simulink model "w2prob4"  (R2020a)
settings: Solver=VariableStepAuto  StartTime=0.0  StopTime=10.0  RelTol=1e-3
PostLoadFcn:
  | J = 3.2284E-6;
  | b = 3.5077E-6;
  | Ke = 0.0274;
  | Kt = 0.0274;
  | R = 4;
  | L = 2.75E-6;
settings Model: DataDictionary=w2p4vars.sldd  Creator=Anjali123  LastModifiedBy=Anjali123

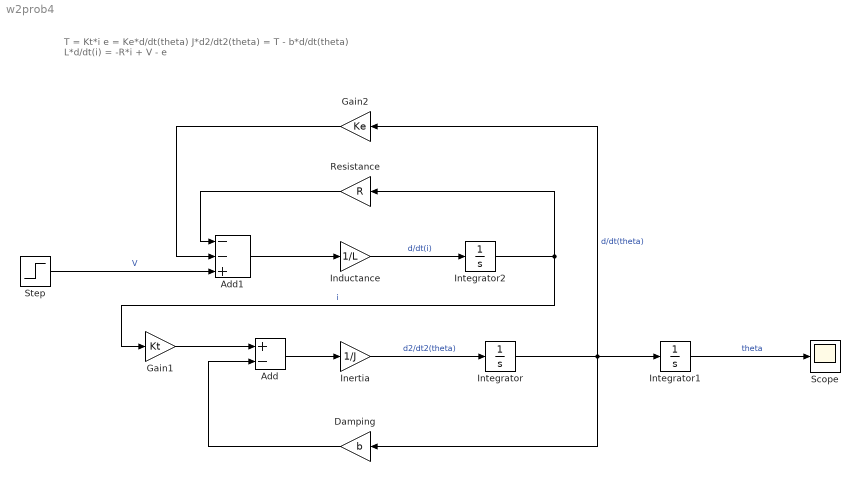
== system w2prob4 ==
  note: T = Kt*i
      | e = Ke*d/dt(theta)
      | J*d2/dt2(theta) = T - b*d/dt(theta)
      | L*d/dt(i) = -R*i + V - e
  "Add " : Sum  Inputs=+-
  "Add1 " : Sum  Inputs=--+
  Damping : Gain  Gain=b
  Gain1 : Gain  Gain=Kt
  Gain2 : Gain  Gain=Ke
  Inductance : Gain  Gain=1/L
  Inertia : Gain  Gain=1/J
  "Integrator " : Integrator
  "Integrator1 " : Integrator
  "Integrator2 " : Integrator
  Resistance : Gain  Gain=R
  Scope : Scope
  Step : Step  SampleTime=0
  wires:
  Inertia/1 -> "Integrator "/1  "d2/dt2(theta)"
  "Integrator "/1 -> Gain2/1, Damping/1, "Integrator1 "/1  "d/dt(theta)"
  "Integrator1 "/1 -> Scope/1  "theta"
  Inductance/1 -> "Integrator2 "/1  "d/dt(i)"
  "Integrator2 "/1 -> Resistance/1, Gain1/1  "i"
  "Add "/1 -> Inertia/1
  "Add1 "/1 -> Inductance/1
  Damping/1 -> "Add "/2
  Gain1/1 -> "Add "/1
  Resistance/1 -> "Add1 "/1
  Gain2/1 -> "Add1 "/2
  Step/1 -> "Add1 "/3  "V"
